simulink model "hierarchical_controller_with_estimator"  (R2024b)
settings: Solver=VariableStepAuto  StartTime=0.0  StopTime=t(end)  RelTol=1e-3
InitFcn:
  | %% UAV PARAMETERS
  | m = 0.5;
  | Ib = diag([0.0023 0.0023 0.00509]);
  | 
  | %% SAMPLING TIME
  | Ts=0.001;
  | 
  | %% TRAJECTORY
  | 
  | % time
  | t = t_tot;
  | 
  | % initial position
  | p0x = points(1,1);
  | p0y = points(1,2);
  | p0z = - points(1,3); % ENU -> NED
  | p0 = [p0x p0y p0z];
  | 
  | % trajectory
  | csi_d=p; dot_csi_d=p_dot; ddot_csi_d=p_ddot;
  | psi_d=zeros(1,length(t)); dot_psi_d=zeros(1,length(t)); ddot_psi_d=zeros(1,length(t));
values from neighbouring files (symbols this model uses):
  K = zeros(1,r)    [filter_coeff.m]
  p = [p segments(i:i+2,:)]    [main_trajectory.m]
  p_ddot = [p_ddot segments_ddot(i:i+2,:)]    [main_trajectory.m]
  p_dot = [p_dot segments_dot(i:i+2,:)]    [main_trajectory.m]
  points = zeros(n,3)    [casual_points.m]    (also in defined_points.m = [0 0 0.2)
  r = 1    [filter_coeff.m]
  t_tot = [t_tot t_temp(i,:)]    [main_trajectory.m]
undefined symbols (not defined in the file or in its folder): ceil_dim, ceil_p, DiscIntNeverNeededParam, par_dim, par_p, supp_dim, support_1_p, support_2_p
libraries: simulink x4, cstblocks x2, dspsigops x2, robotcorelib x1, uavutilslib x1
settings Model: Creator=ricca  LastModifiedBy=ricca

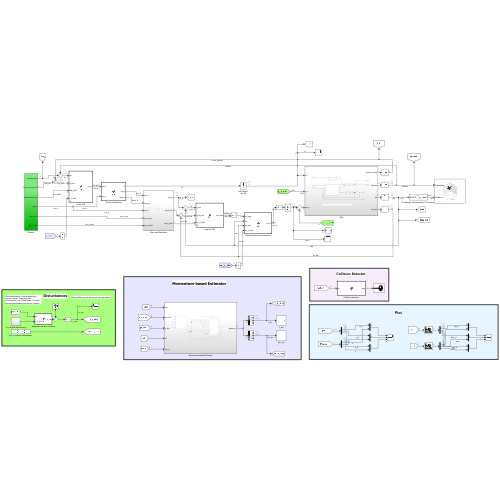
[thumbnail: Simulink's stored preview of the top-level diagram]
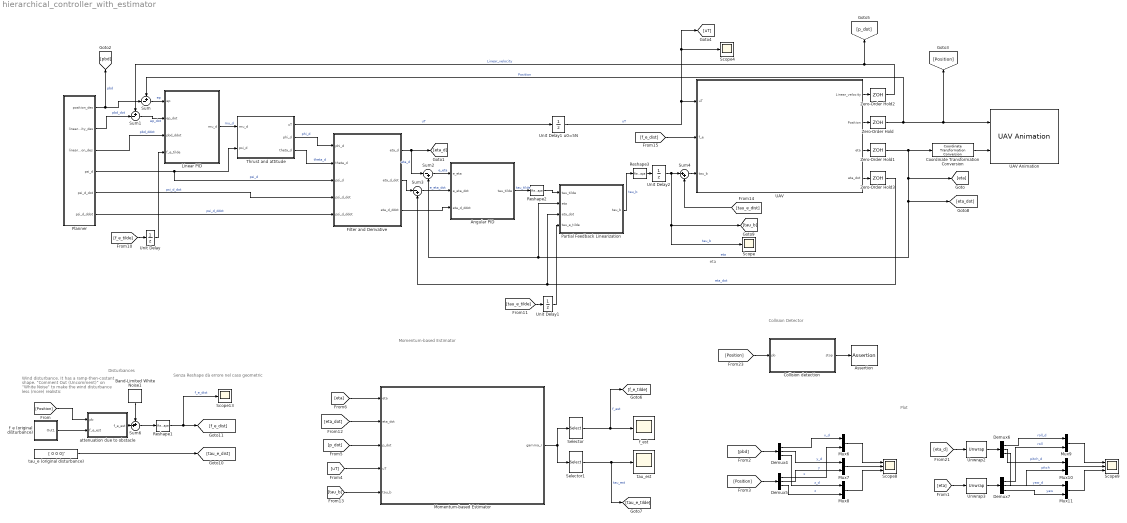
== system hierarchical_controller_with_estimator ==
  note: eta
  note: Momentum-based Estimator
  note: Collision Detector
  note: Plot
  note: Senza Reshape dà errore nel caso geometric
  note: Disturbances
  note: Wind disturbance. It has a ramp-then-costant shape. "Comment Out (Uncomment)" on "White Noise" to make the wind disturbance less (more) realistic
  Angular PID : MATLAB Function  TreatAsAtomicUnit=on  mask(Angular PID){Ke=[100*eye(3) 100*eye(3)]}
      mask help: Ke ∈ R^(3x6)
  Assertion : Assertion  AssertionFailFcn='WARNING: DRONE CRASHED!'
  Band-Limited White Noise1 : simulink/Sources/Band-Limited White Noise  Cov=[0.0001 0.0001 0]'  Ts=0.1  seed=[23341 23345 0]'  VectorParams1D=off
  Collision detection : MATLAB Function  TreatAsAtomicUnit=on
  Coordinate Transformation Conversion : robotcorelib/Coordinate Transformation Conversion  InputRepresentation=Euler Angles  InputEulerSequence=XYZ  ShowTrVecInputPort=on  OutputRepresentation=Quaternion  OutputEulerSequence=ZYX  ShowTrVecOutputPort=on  SimulateUsing=Interpreted execution
  Demux{4..7} (4 alike) : Demux  Outputs=3
  Filter and Derivative : Subsystem
  Linear PID : MATLAB Function  TreatAsAtomicUnit=on  mask(Position PID){Kp=[10*eye(3) 10*eye(3)]}
      mask help: Kp ∈ R^(3x6)
  Momentum-based Estimator : Subsystem
  Mux{6..11} (6 alike) : Mux  Inputs=2
  Partial Feedback Linearization : MATLAB Function  TreatAsAtomicUnit=on
  Planner : Subsystem
  Reshape1 : Reshape
  Reshape2 : Reshape
  Reshape3 : Reshape
  Scope : Scope
  Scope13 : Scope
  Scope4 : Scope
  Scope8 : Scope  NumInputPorts=3
  Scope9 : Scope  NumInputPorts=3
  Selector : Selector  InputPortWidth=6  IndexOptions=Index vector (dialog)  Indices=[1 2 3]  OutputSizes=1
  Selector1 : Selector  InputPortWidth=6  IndexOptions=Index vector (dialog)  Indices=[4 5 6]  OutputSizes=1
  Sum : Sum  Inputs=+-|
  Sum1 : Sum  Inputs=+-|
  Sum2 : Sum  Inputs=|-+
  Sum3 : Sum  Inputs=|-+
  Sum4 : Sum  Inputs=|++
  Sum6 : Sum  Inputs=++|
  Thrust and attitude : MATLAB Function  TreatAsAtomicUnit=on
  UAV : Subsystem
  UAV Animation : uavutilslib/UAV Animation  NumUAV=1  DynamicUAVConfig=off  UAVType=Multirotor  UAVSize=1  UAVColor=[1 0 0]  UAVTrajectoryAlpha=1  InertialZDirection=Down  RotationFormat=Quaternion  DrawMarkers=off  SampleTime=-1
  Unit Delay : UnitDelay  SampleTime=Ts  HasFrameUpgradeWarning=on
  Unit Delay1 : UnitDelay  SampleTime=Ts  HasFrameUpgradeWarning=on
  Unit Delay1 u0=5N : UnitDelay  InitialCondition=5  SampleTime=Ts
  Unit Delay2 : UnitDelay  InitialCondition=[0 0 0]  SampleTime=Ts
  Unwrap2 : dspsigops/Unwrap  tol=pi  InputProcessing=Columns as channels (frame based)  running=off
  Unwrap3 : dspsigops/Unwrap  tol=pi  InputProcessing=Columns as channels (frame based)  running=off
  Zero-Order Hold{,1..3} (4 alike) : ZeroOrderHold  SampleTime=-1
  attenuation due to obstacle : MATLAB Function  TreatAsAtomicUnit=on
  f_e (original disturbance) : Subsystem
  f_est : Scope
  tau_e (original disturbance) : Constant  Value=[ 0 0 0]'
  tau_est : Scope
  wires:
  Zero-Order Hold1/1 -> Coordinate Transformation Conversion/1, [eta_dot], Sum2/2, Partial Feedback Linearization/2(eta), [eta]  "eta"
  Coordinate Transformation Conversion/1 -> UAV Animation/2
  Thrust and attitude/1(uT) -> Unit Delay1 u0=5N/1  "uT"
  Linear PID/1(mu_d) -> Thrust and attitude/1(mu_d)  "mu_d"
  Zero-Order Hold/1 -> Sum/1, UAV Animation/1, [Position]  "Position"
  Sum/1 -> Linear PID/1(ep)  "ep"
  Planner/1(position_des) -> Sum/2, [pbd]  "pbd"
  Zero-Order Hold2/1 -> Sum1/1, [p_dot]  "Linear_velocity"
  Planner/2(linear_velocity_des) -> Sum1/2  "pbd_dot"
  Sum1/1 -> Linear PID/2(ep_dot)  "ep_dot"
  Planner/3(linear_acceleration_des) -> Linear PID/3(pbd_ddot)  "pbd_ddot"
  Planner/4(psi_d) -> Filter and Derivative/3(psi_d), Thrust and attitude/2(psi_d)  "psi_d"
  Angular PID/1(tau_tilde) -> Reshape2/1  "tau_tilde"
  Sum2/1 -> Angular PID/1(e_eta)  "e_eta"
  Sum3/1 -> Angular PID/2(e_eta_dot)  "e_eta_dot"
  Planner/5(psi_d_dot) -> Filter and Derivative/4(psi_d_dot)  "psi_d_dot"
  Planner/6(psi_d_ddot) -> Filter and Derivative/5(psi_d_ddot)  "psi_d_ddot"
  Thrust and attitude/2(phi_d) -> Filter and Derivative/1(phi_d)  "phi_d"
  Thrust and attitude/3(theta_d) -> Filter and Derivative/2(theta_d)  "theta_d"
  Filter and Derivative/2(eta_d_dot) -> Sum3/1
  Filter and Derivative/3(eta_d_ddot) -> Angular PID/3(eta_d_ddot)
  Reshape3/1 -> Unit Delay2/1
  Unit Delay2/1 -> Scope/1, [tau_b], Sum4/1  "tau_b"
  UAV/1(Linear_velocity) -> Zero-Order Hold2/1
  UAV/2(Position) -> Zero-Order Hold/1
  UAV/3(eta) -> Zero-Order Hold1/1
  UAV/4(eta_dot) -> Zero-Order Hold3/1
  Unit Delay1 u0=5N/1 -> [uT], Scope4/1, UAV/1(uT)  "uT"
  Filter and Derivative/1(eta_d) -> [eta_d], Sum2/1  "eta_d"
  Partial Feedback Linearization/1(tau_b) -> Reshape3/1  "tau_b"
  Zero-Order Hold3/1 -> Sum3/2, Partial Feedback Linearization/3(eta_dot)  "eta_dot"
  Sum4/1 -> UAV/3(tau_b)
  Reshape2/1 -> Partial Feedback Linearization/1(tau_tilde)
  [f_e_tilde] -> Unit Delay/1
  Unit Delay/1 -> Linear PID/4(f_e_tilde)
  [tau_e_tilde] -> Unit Delay1/1
  Unit Delay1/1 -> Partial Feedback Linearization/4(tau_e_tilde)
  [tau_e_dist] -> Sum4/2
  [f_e_dist] -> UAV/2(f_e)
  [uT] -> Momentum-based Estimator/4(uT)
  [eta] -> Momentum-based Estimator/1(eta)
  Selector1/1 -> [tau_e_tilde], tau_est/1  "tau_est"
  Selector/1 -> [f_e_tilde], f_est/1  "f_est"
  [tau_b] -> Momentum-based Estimator/5(tau_b)
  [eta_dot] -> Momentum-based Estimator/2(eta_dot)
  [p_dot] -> Momentum-based Estimator/3(p_dot)
  Momentum-based Estimator/1(gamma_r) -> Selector/1, Selector1/1
  Demux6/2 -> Mux10/1  "pitch_d"
  Demux4/3 -> Mux8/1  "z_d"
  Demux4/2 -> Mux7/1  "y_d"
  Demux4/1 -> Mux6/1  "x_d"
  Collision detection/1(stop) -> Assertion/1
  Mux11/1 -> Scope9/3
  Unwrap3/1 -> Demux7/1
  [Position] -> Collision detection/1(pb)
  Demux6/1 -> Mux9/1  "roll_d"
  [eta] -> Unwrap3/1
  Demux5/1 -> Mux6/2  "x"
  Demux7/2 -> Mux10/2  "pitch"
  Mux8/1 -> Scope8/3
  Demux5/3 -> Mux8/2  "z"
  Demux6/3 -> Mux11/1  "yaw_d"
  Mux6/1 -> Scope8/1
  [Position] -> Demux5/1
  Demux7/1 -> Mux9/2  "roll"
  Mux9/1 -> Scope9/1
  [eta_d] -> Unwrap2/1
  Mux10/1 -> Scope9/2
  Demux7/3 -> Mux11/2  "yaw"
  [pbd] -> Demux4/1
  Mux7/1 -> Scope8/2
  Unwrap2/1 -> Demux6/1
  Demux5/2 -> Mux7/2  "y"
  attenuation due to obstacle/1(f_e_est) -> Sum6/2
  f_e (original disturbance)/1(Out1) -> attenuation due to obstacle/2("f_e_est ")
  Sum6/1 -> Reshape1/1
  Reshape1/1 -> Scope13/1, [f_e_dist]  "f_e_dist"
  [Position] -> attenuation due to obstacle/1(pb)
  Band-Limited White Noise1/1 -> Sum6/1
  tau_e (original disturbance)/1 -> [tau_e_dist]

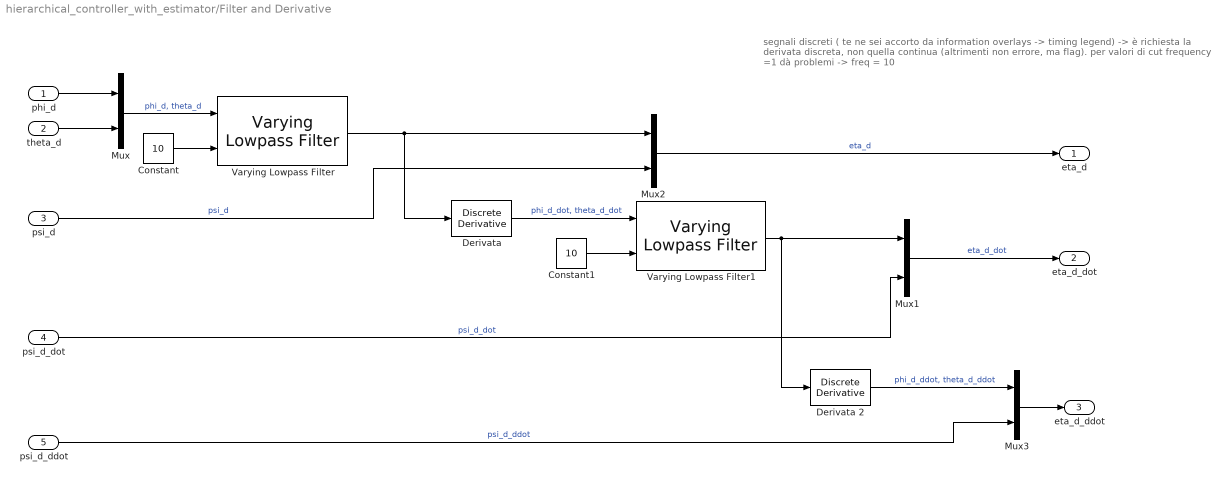
== system hierarchical_controller_with_estimator/Filter and Derivative ==
  note: segnali discreti ( te ne sei accorto da information overlays -> timing legend) -> è richiesta la derivata discreta, non quella continua (altrimenti non errore, ma flag).
      |
      | per valori di cut frequency =1 dà problemi -> freq = 10
  phi_d : Inport
  theta_d : Inport  Port=2
  psi_d : Inport  Port=3
  psi_d_dot : Inport  Port=4
  psi_d_ddot : Inport  Port=5
  Constant : Constant  Value=10
  Constant1 : Constant  Value=10
  Derivata : simulink/Discrete/Discrete Derivative  gainval=1.0  ICPrevScaledInput=0.0  OutMin=[]  OutMax=[]  OutDataType=fixdt(1, 16)  OutScaling=2^-10  DoSatur=off
  Derivata 2 : simulink/Discrete/Discrete Derivative  gainval=1.0  ICPrevScaledInput=0.0  OutMin=[]  OutMax=[]  OutDataType=fixdt(1, 16)  OutScaling=2^-10  DoSatur=off
  Mux{,1..3} (4 alike) : Mux  Inputs=2
  Varying Lowpass Filter : cstblocks/Linear Parameter Varying/Varying Lowpass Filter  N=1
  Varying Lowpass Filter1 : cstblocks/Linear Parameter Varying/Varying Lowpass Filter  N=1
  eta_d : Outport
  eta_d_dot : Outport  Port=2
  eta_d_ddot : Outport  Port=3
  wires:
  Derivata/1 -> Varying Lowpass Filter1/1  "phi_d_dot, theta_d_dot"
  theta_d/1 -> Mux/2
  phi_d/1 -> Mux/1
  psi_d/1 -> Mux2/2  "psi_d"
  Mux2/1 -> eta_d/1  "eta_d"
  psi_d_dot/1 -> Mux1/2  "psi_d_dot"
  Mux1/1 -> eta_d_dot/1  "eta_d_dot"
  Mux3/1 -> eta_d_ddot/1
  Derivata 2/1 -> Mux3/1  "phi_d_ddot, theta_d_ddot"
  psi_d_ddot/1 -> Mux3/2  "psi_d_ddot"
  Mux/1 -> Varying Lowpass Filter/1  "phi_d, theta_d"
  Varying Lowpass Filter/1 -> Derivata/1, Mux2/1
  Constant/1 -> Varying Lowpass Filter/2
  Varying Lowpass Filter1/1 -> Derivata 2/1, Mux1/1
  Constant1/1 -> Varying Lowpass Filter1/2

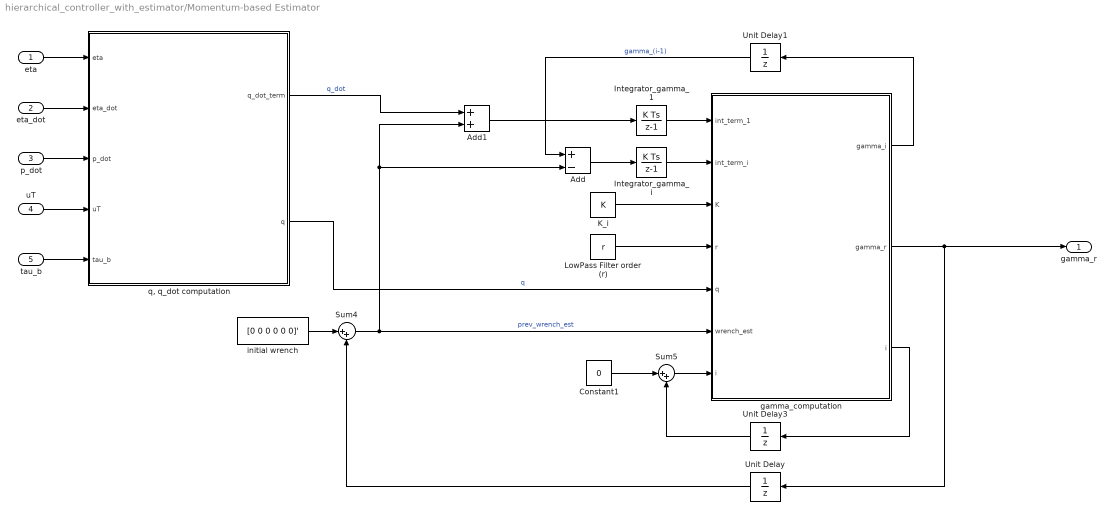
== system hierarchical_controller_with_estimator/Momentum-based Estimator ==
  eta : Inport
  eta_dot : Inport  Port=2
  p_dot : Inport  Port=3
  uT : Inport  Port=4
  tau_b : Inport  Port=5
  Add : Sum  Inputs=+-
  Add1 : Sum
  Constant1 : Constant  Value=0
  Integrator_gamma_1 : DiscreteIntegrator  SampleTime=Ts  ICPrevOutput=DiscIntNeverNeededParam  ICPrevScaledInput=DiscIntNeverNeededParam
  Integrator_gamma_i : DiscreteIntegrator  SampleTime=Ts  ICPrevOutput=DiscIntNeverNeededParam  ICPrevScaledInput=DiscIntNeverNeededParam
  K_i : Constant  Value=K
  LowPass Filter order (r) : Constant  Value=r
  Sum4 : Sum  Inputs=|++
  Sum5 : Sum  Inputs=|++
  Unit Delay : UnitDelay  SampleTime=Ts  HasFrameUpgradeWarning=on
  Unit Delay1 : UnitDelay  SampleTime=Ts  HasFrameUpgradeWarning=on
  Unit Delay3 : UnitDelay  SampleTime=Ts  HasFrameUpgradeWarning=on
  gamma_computation : MATLAB Function  TreatAsAtomicUnit=on
  initial wrench : Constant  Value=[0 0 0 0 0 0]'
  "q, q_dot computation" : MATLAB Function  TreatAsAtomicUnit=on
  gamma_r : Outport
  wires:
  Unit Delay/1 -> Sum4/2
  p_dot/1 -> "q, q_dot computation"/3(p_dot)
  LowPass Filter order (r)/1 -> gamma_computation/4(r)
  Sum4/1 -> gamma_computation/6(wrench_est), Add/2, Add1/2  "prev_wrench_est"
  gamma_computation/2(gamma_r) -> Unit Delay/1, gamma_r/1
  Add1/1 -> Integrator_gamma_1/1
  Add/1 -> Integrator_gamma_i/1
  Unit Delay1/1 -> Add/1  "gamma_(i-1)"
  gamma_computation/1(gamma_i) -> Unit Delay1/1
  Constant1/1 -> Sum5/1
  uT/1 -> "q, q_dot computation"/4(uT)
  "q, q_dot computation"/1(q_dot_term) -> Add1/1  "q_dot"
  K_i/1 -> gamma_computation/3(K)
  initial wrench/1 -> Sum4/1
  Integrator_gamma_1/1 -> gamma_computation/1(int_term_1)
  "q, q_dot computation"/2(q) -> gamma_computation/5(q)  "q"
  Sum5/1 -> gamma_computation/7("i ")
  Integrator_gamma_i/1 -> gamma_computation/2(int_term_i)
  gamma_computation/3(i) -> Unit Delay3/1
  Unit Delay3/1 -> Sum5/2
  eta_dot/1 -> "q, q_dot computation"/2(eta_dot)
  tau_b/1 -> "q, q_dot computation"/5(tau_b)
  eta/1 -> "q, q_dot computation"/1(eta)

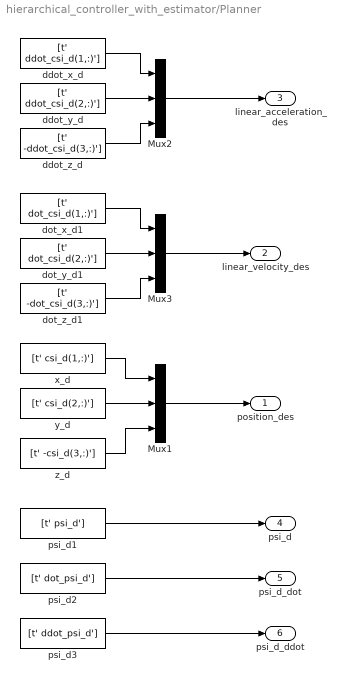
== system hierarchical_controller_with_estimator/Planner ==
  Mux1 : Mux  Inputs=3
  Mux2 : Mux  Inputs=3
  Mux3 : Mux  Inputs=3
  ddot_x_d : FromWorkspace  VariableName=[t' ddot_csi_d(1,:)']  SampleTime=Ts
  ddot_y_d : FromWorkspace  VariableName=[t' ddot_csi_d(2,:)']  SampleTime=Ts
  ddot_z_d : FromWorkspace  VariableName=[t' -ddot_csi_d(3,:)']  SampleTime=Ts
  dot_x_d1 : FromWorkspace  VariableName=[t' dot_csi_d(1,:)']  SampleTime=Ts
  dot_y_d1 : FromWorkspace  VariableName=[t' dot_csi_d(2,:)']  SampleTime=Ts
  dot_z_d1 : FromWorkspace  VariableName=[t' -dot_csi_d(3,:)']  SampleTime=Ts
  psi_d1 : FromWorkspace  VariableName=[t' psi_d']  SampleTime=Ts
  psi_d2 : FromWorkspace  VariableName=[t' dot_psi_d']  SampleTime=Ts
  psi_d3 : FromWorkspace  VariableName=[t' ddot_psi_d']  SampleTime=Ts
  x_d : FromWorkspace  VariableName=[t' csi_d(1,:)']  SampleTime=Ts
  y_d : FromWorkspace  VariableName=[t' csi_d(2,:)']  SampleTime=Ts
  z_d : FromWorkspace  VariableName=[t' -csi_d(3,:)']  SampleTime=Ts
  position_des : Outport
  linear_velocity_des : Outport  Port=2
  linear_acceleration_des : Outport  Port=3
  psi_d : Outport  Port=4
  psi_d_dot : Outport  Port=5
  psi_d_ddot : Outport  Port=6
  wires:
  y_d/1 -> Mux1/2
  z_d/1 -> Mux1/3
  x_d/1 -> Mux1/1
  ddot_y_d/1 -> Mux2/2
  ddot_z_d/1 -> Mux2/3
  ddot_x_d/1 -> Mux2/1
  Mux2/1 -> linear_acceleration_des/1
  Mux1/1 -> position_des/1
  dot_y_d1/1 -> Mux3/2
  dot_z_d1/1 -> Mux3/3
  dot_x_d1/1 -> Mux3/1
  Mux3/1 -> linear_velocity_des/1
  psi_d1/1 -> psi_d/1
  psi_d2/1 -> psi_d_dot/1
  psi_d3/1 -> psi_d_ddot/1

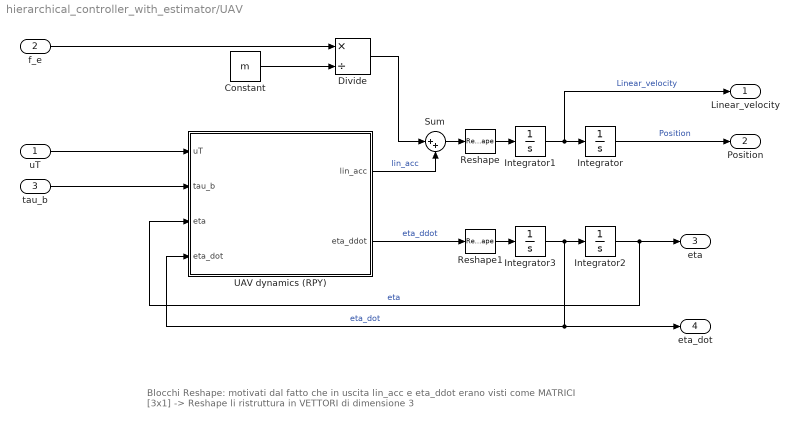
== system hierarchical_controller_with_estimator/UAV ==
  note: Blocchi Reshape: motivati dal fatto che in uscita lin_acc e eta_ddot erano visti come MATRICI [3x1] -> Reshape li ristruttura in VETTORI di dimensione 3
  uT : Inport
  f_e : Inport  Port=2
  tau_b : Inport  Port=3
  Constant : Constant  Value=m
  Divide : Product  Inputs=*/
  Integrator : Integrator  InitialCondition=p0
  Integrator1 : Integrator  InitialCondition=[0 0 0]
  Integrator2 : Integrator  InitialCondition=[0 0 0]
  Integrator3 : Integrator  InitialCondition=[0 0 0]
  Reshape : Reshape
  Reshape1 : Reshape
  Sum : Sum  Inputs=|++
  UAV dynamics (RPY) : MATLAB Function  TreatAsAtomicUnit=on
  Linear_velocity : Outport
  Position : Outport  Port=2
  eta : Outport  Port=3
  eta_dot : Outport  Port=4
  wires:
  Integrator2/1 -> eta/1, UAV dynamics (RPY)/3(eta)  "eta"
  UAV dynamics (RPY)/1(lin_acc) -> Sum/2  "lin_acc"
  Integrator1/1 -> Linear_velocity/1, Integrator/1  "Linear_velocity"
  Integrator3/1 -> eta_dot/1, UAV dynamics (RPY)/4(eta_dot), Integrator2/1  "eta_dot"
  Reshape1/1 -> Integrator3/1
  Reshape/1 -> Integrator1/1
  UAV dynamics (RPY)/2(eta_ddot) -> Reshape1/1  "eta_ddot"
  uT/1 -> UAV dynamics (RPY)/1(uT)
  tau_b/1 -> UAV dynamics (RPY)/2(tau_b)
  Integrator/1 -> Position/1  "Position"
  f_e/1 -> Divide/1
  Sum/1 -> Reshape/1
  Constant/1 -> Divide/2
  Divide/1 -> Sum/1

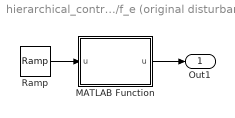
== system hierarchical_controller_with_estimator/f_e (original disturbance) ==
  MATLAB Function : MATLAB Function  TreatAsAtomicUnit=on
  Ramp : simulink/Sources/Ramp  slope=[ 0.1 0.1 0]'  start=5  InitialOutput=0  VectorParams1D=off
  Out1 : Outport
  wires:
  Ramp/1 -> MATLAB Function/1("u ")
  MATLAB Function/1(u) -> Out1/1

== matlab function hierarchical_controller_with_estimator/attenuation due to obstacle ==
  data: pb input; f_e_est input; f_e_est output; ceil_dim parameter; ceil_p parameter; supp_dim parameter
function f_e_est = fcn(pb,f_e_est,ceil_dim, ceil_p, supp_dim)

% quadrotor coordinates
x = pb(1);
y = pb(2);
z = pb(3); % ricordare che ha segno negativo (NED frame)

% OCCHIO: ricordare che nella configurazione NED le z sono NEGATIVE!!!
% Quindi devi ragionare al contrario per le condizioni di passaggio
% nell'ostacolo

% CONDIZIONE PASSAGGIO ALL'INTERNO DEL PRIMO OSTACOLO
if       x >= ceil_p(1) - ceil_dim(1)/2                  &&   x <= ceil_p(1) + ceil_dim(1)/2                    && ...
         y >= ceil_p(2) - (ceil_dim(2)/2 - supp_dim(2))  &&   y <= ceil_p(2) + (ceil_dim(2)/2 - supp_dim(2))    && ...
         z >= -supp_dim(3)                               &&   z <= 0
    
    if f_e_est(2) >= 0.1            % Se c'è vento moderato lungo l'asse y ...
        f_e_est(2) = f_e_est(2)/2;  % ...dimezzo la sua intensità lungo tale asse, perché impatta contro il supporto dell'ostacolo.
    else                            % Se il vento è di bassa intensità lungo l'asse y ...
        f_e_est(2) = 0;             % l'impatto con il support blocca completamente il vento lungo tale asse. 
    end
end

end

== matlab function hierarchical_controller_with_estimator/Collision detection ==
  data: pb input; stop output; ceil_p parameter; par_p parameter; ceil_dim parameter; par_dim parameter; supp_dim parameter; support_1_p parameter; support_2_p parameter
function stop =  f(pb, ceil_p, par_p, ceil_dim, par_dim, supp_dim, support_1_p, support_2_p)

% OCCHIO: le dimensioni degli ostacoli e le dimensioni x e y della posizione
% del drone sono positive. La dimensione z del drone NO: sono negative 
% (NED frame)! Attento nelle formule e nelle condizioni dei costrutti 
% if/else

% Dovrò tenere in conto anche della mesh del drone:

% ** Maximum width with propeller = 0.57 m -> maximum radius with propeller = 0.285 m
r = 0.285;

% ** Height = 0.1 m -> distance "center of mass - upper/lower" tip = 0.05 m
h = 0.05;

%% INITIALIZATION
stop = 1; % if no collision -> stop = 1

x = pb(1);
y = pb(2);
z = pb(3); % it is a negative value because of the NED configuration


%% COLLISION DETECTION
% if there is a collision -> stop = 0 

% Collision with the ground
if              z >= 0 - h
    stop = 0;

% Collision with the ceiling
elseif          x >= ceil_p(1) - ceil_dim(1)/2 - r                  &&   x <= ceil_p(1) + ceil_dim(1)/2 + r               && ... % le condizioni sull'asse x sono state fatte rispetto alla posizione del centro e alle dimensioni rispetto a x del soffitto
                y >= ceil_p(2) - ceil_dim(2)/2 - r                  &&   y <= ceil_p(2) + ceil_dim(2)/2 + r               && ... % le condizioni sull'asse y sono state fatte rispetto alla posizione del centro e alle dimensioni rispetto a y del soffitto
                z <= -supp_dim(3) + h                               &&   z >= -(supp_dim(3) + ceil_dim(3)) - h                   % le condizioni sull'asse z sono state fatte rispetto all'altezza dei sostegni (supposti uguali) + lo spessore del soffitto (dimensione in z)

    stop = 0; % STOP VALUE

% Collision with the 1st ceiling support
elseif          x >= support_1_p(1) - supp_dim(1)/2 - r             &&   x <= support_1_p(1) + supp_dim(1)/2 + r          && ... % le condizioni sull'asse x sono state fatte rispetto alla posizione del centro e alle dimensioni rispetto a x del primo supporto (con supporti supposti uguali)
                y >= support_1_p(2) - supp_dim(2)/2 - r             &&   y <= support_1_p(2) + supp_dim(2)/2 + r          && ... % le condizioni sull'asse y sono state fatte rispetto alla posizione del centro e alle dimensioni rispetto a y del primo supporto (con supporti supposti uguali)
                z <= 0 + h                                          &&   z >= -supp_dim(3) - h                                   % le condizioni sull'asse z sono state fatte rispetto all'altezza dei sostegni (supposti uguali) + lo spessore del soffitto (dimensione in z)

    stop = 0; % STOP VALUE

% Collision with the 2nd ceiling support
elseif          x >= support_2_p(1) - supp_dim(1)/2 - r             &&   x <= support_2_p(1) + supp_dim(1)/2 + r          && ... % le condizioni sull'asse x sono state fatte rispetto alla posizione del centro e alle dimensioni rispetto a x del secondo supporto (con supporti supposti uguali)
                y >= support_2_p(2) - supp_dim(2)/2 - r             &&   y <= support_2_p(2) + supp_dim(2)/2 + r          && ... % le condizioni sull'asse y sono state fatte rispetto alla posizione del centro e alle dimensioni rispetto a y del secondo supporto (con supporti supposti uguali)
                z <= 0 + h                                          &&   z >= -supp_dim(3) - h                                   % le condizioni sull'asse z sono state fatte rispetto all'altezza dei sostegni (supposti uguali) + lo spessore del soffitto (dimensione in z)

    stop = 0; % STOP VALUE

% Collision with the  parallelepiped
elseif          x >= par_p(1) - par_dim(1)/2 - r                    &&   x <= par_p(1) + par_dim(1)/2 + r                  && ... % le condizioni sull'asse x sono state fatte rispetto alla posizione del centro e alle dimensioni rispetto a x della colonna (parallelepipedo)
                y >= par_p(2) - par_dim(2)/2 - r                    &&   y <= par_p(2) + par_dim(2)/2 + r                  && ... % le condizioni sull'asse y sono state fatte rispetto alla posizione del centro e alle dimensioni rispetto a y della colonna (parallelepipedo)
                z <= 0 + h                                          &&   z >= -par_dim(3) - h                                     % le condizioni sull'asse z sono state fatte rispetto all'altezza della colonna partendo dal pavimento (dimensione in z)

    stop = 0; % STOP VALUE

end

end

== matlab function hierarchical_controller_with_estimator/f_e (original disturbance)/MATLAB Function ==
  data: u input; u output
function u = fcn(u)
if u >= [0.1 0.1 0]'
    u = [0.1 0.1 0]';
end

== matlab function hierarchical_controller_with_estimator/Thrust and attitude ==
  data: mu_d input; uT output; phi_d output; theta_d output; psi_d input; m parameter
function [uT, phi_d, theta_d] = fcn(mu_d,psi_d,m)

uT = m*sqrt( mu_d(1)^2 + mu_d(2)^2 + (mu_d(3)-9.81)^2 );
phi_d = asin(m/uT*(mu_d(2)*cos(psi_d) - mu_d(1)*sin(psi_d)));
theta_d = atan((mu_d(1)*cos(psi_d) + mu_d(2)*sin(psi_d))/(mu_d(3)-9.81));

end

== matlab function hierarchical_controller_with_estimator/UAV/UAV dynamics (RPY) ==
  data: uT input; lin_acc output; tau_b input; eta input; eta_dot input; eta_ddot output; Ib parameter; m parameter
function [lin_acc, eta_ddot] = fcn(uT,tau_b, eta,eta_dot,Ib, m)

phi = eta(1);
theta = eta(2);
psi = eta(3);

phi_dot = eta_dot(1);
theta_dot = eta_dot(2);
psi_dot = eta_dot(3);

% Rb
Rb = [cos(theta)*cos(psi)    sin(phi)*sin(theta)*cos(psi) - cos(phi)*sin(psi)     cos(phi)*sin(theta)*cos(psi) + sin(phi)*sin(psi);
      cos(theta)*sin(psi)    sin(phi)*sin(theta)*sin(psi) + cos(phi)*cos(psi)     cos(phi)*sin(theta)*sin(psi) - sin(phi)*cos(psi);
          -sin(theta)                     sin(phi)*cos(theta)                                 cos(phi)*cos(theta)                ];

% Q(eta)
Q = [1          0       -sin(theta);
     0      cos(phi)     cos(theta)*sin(phi);
     0     -sin(phi)     cos(theta)*cos(phi)];

% Q_dot(eta)
Q_dot = [0        0                 cos(theta)*theta_dot;
         0    -sin(phi)*phi_dot    -sin(theta)*theta_dot*sin(phi) + cos(theta)*cos(phi)*phi_dot;
         0    -cos(phi)*phi_dot    -sin(theta)*theta_dot*cos(phi) - cos(theta)*sin(phi)*phi_dot];

% M(eta)
M = Q'*Ib*Q;

% C(eta,eta_dot)
C = Q'*skew(Q*eta_dot)*Ib*Q + Q'*Ib*Q_dot;


% RPY dynamic model 
lin_acc = 9.81*[0 0 1]'-(uT/m)*Rb*[0 0 1]';
eta_ddot = inv(M)*(-C*eta_dot + Q'*tau_b);

end


function S = skew(v)
if (numel(v)~= 1)
    S= [0 -v(3) v(2);
        v(3) 0 -v(1);
        -v(2) v(1) 0];
else
    S= zeros(3);
end
end

== matlab function hierarchical_controller_with_estimator/Linear PID ==
  data: ep input; mu_d output; ep_dot input; pbd_ddot input; f_e_tilde input; m parameter; Kp parameter
function mu_d = fcn(ep,ep_dot,pbd_ddot,f_e_tilde,m,Kp)

mu_d = -Kp*[ep;ep_dot] + pbd_ddot - f_e_tilde/m;

% acceleration handling
if mu_d(3) >= 9.81
    mu_d(3) = 9.8;
elseif mu_d(3) <= -9.81
    mu_d(3) = -9.8;
end


end

== matlab function hierarchical_controller_with_estimator/Partial Feedback Linearization ==
  data: tau_b output; tau_tilde input; eta input; eta_dot input; Ib parameter; tau_e_tilde input
function tau_b = fcn(tau_tilde,eta,eta_dot, Ib, tau_e_tilde)

phi = eta(1);
theta = eta(2);
psi = eta(3);

phi_dot = eta_dot(1);
theta_dot = eta_dot(2);
psi_dot = eta_dot(3);


% Q(eta)
Q = [1          0       -sin(theta);
     0      cos(phi)     cos(theta)*sin(phi);
     0     -sin(phi)     cos(theta)*cos(phi)];

% Q_dot(eta)
Q_dot = [0        0                 cos(theta)*theta_dot;
         0    -sin(phi)*phi_dot    -sin(theta)*theta_dot*sin(phi) + cos(theta)*cos(phi)*phi_dot;
         0    -cos(phi)*phi_dot    -sin(theta)*theta_dot*cos(phi) - cos(theta)*sin(phi)*phi_dot];

% C(eta,eta_dot)
C = Q'*skew(Q*eta_dot)*Ib*Q + Q'*Ib*Q_dot;

% tau_b
tau_b = Ib*Q*tau_tilde  + inv(Q')*C*eta_dot - inv(Q')*tau_e_tilde;

end


function S = skew(v)
if (numel(v)~= 1)
    S= [0 -v(3) v(2);
        v(3) 0 -v(1);
        -v(2) v(1) 0];
else
    S= zeros(3);
end
end

== matlab function hierarchical_controller_with_estimator/Angular PID ==
  data: e_eta input; e_eta_dot input; eta_d_ddot input; tau_tilde output; Ke parameter
function tau_tilde = fcn(e_eta,e_eta_dot,eta_d_ddot,Ke)

tau_tilde = -Ke*[e_eta;e_eta_dot] + eta_d_ddot;

end

== matlab function hierarchical_controller_with_estimator/Momentum-based Estimator/gamma_computation ==
  data: int_term_1 input; int_term_i input; K input; r input; q input; wrench_est input; gamma_i output; gamma_r output; i input; i output
function [gamma_i,gamma_r, i] = fcn(int_term_1, int_term_i,K,r,q, wrench_est, i)
gamma_r = wrench_est;
gamma_i = zeros(6,1);

if r == 1 % quando è di ordine 1
    gamma_i = K(1)*eye(6)*(q-int_term_1);  % infatti i coefficienti riguardano il i-esimo filtro Gi(s) con i = 1,...,6. Quindi abbiamo 6 coefficienti per i 6 filtri
    gamma_r = gamma_i;
else % quando l'ordine è maggiore di 1
    if i == 0
        i = i+1;
        gamma_i = K(1)*eye(6)*(q-int_term_1);
    else
        i = i+1;
        gamma_i = K(i)*eye(6)*int_term_i;
        if i == r
            gamma_r = gamma_i;
            i = 0;
        end
    end
end

end

== matlab function hierarchical_controller_with_estimator/Momentum-based Estimator/q, q_dot computation ==
  data: eta input; eta_dot input; p_dot input; uT input; q_dot_term output; q output; tau_b input; Ib parameter; m parameter
function [q_dot_term, q] = fcn(eta, eta_dot,p_dot,uT,tau_b,Ib,m)

e_3 = [0 0 1]';
g = 9.81;
I3 = eye(3);
O3 = zeros(3);

phi = eta(1);
theta = eta(2);
psi = eta(3);

phi_dot = eta_dot(1);
theta_dot = eta_dot(2);
psi_dot = eta_dot(3);


% Q(eta)
Q = [1          0       -sin(theta);
     0      cos(phi)     cos(theta)*sin(phi);
     0     -sin(phi)     cos(theta)*cos(phi)];

% Q_dot(eta)
Q_dot = [0        0                 cos(theta)*theta_dot;
         0    -sin(phi)*phi_dot    -sin(theta)*theta_dot*sin(phi) + cos(theta)*cos(phi)*phi_dot;
         0    -cos(phi)*phi_dot    -sin(theta)*theta_dot*cos(phi) - cos(theta)*sin(phi)*phi_dot];

% C(eta,eta_dot)
C = Q'*skew(Q*eta_dot)*Ib*Q + Q'*Ib*Q_dot;

% M(eta)
M = Q'*Ib*Q;

%Rb
Rb = [cos(theta)*cos(psi) (sin(phi)*sin(theta)*cos(psi)-cos(phi)*sin(psi)) (cos(phi)*sin(theta)*cos(psi)+sin(phi)*sin(psi));
      cos(theta)*sin(psi) (sin(phi)*sin(theta)*sin(psi)+cos(phi)*cos(psi)) (cos(phi)*sin(theta)*sin(psi)-sin(phi)*cos(psi));
      -sin(theta) sin(phi)*cos(theta) cos(phi)*cos(theta)];

%%% OUTPUT
q = [m*I3 O3; O3 M]*[p_dot;eta_dot];
q_dot_term = [m*g*e_3 - uT*Rb*e_3; C'*eta_dot + Q'*tau_b];

end



function S = skew(v)
if (numel(v)~= 1)
    S= [0 -v(3) v(2);
        v(3) 0 -v(1);
        -v(2) v(1) 0];
else
    S= zeros(3);
end
end
